simulink model "Openloop_SMA_wire_param"  (R2016b)
settings: Solver=FixedStepAuto  StartTime=0.0  StopTime=20  FixedStep=0.00001  MinStep=0.0001  RelTol=1e-3
values from neighbouring files (symbols this model uses):
  Ac = (pi*d^2)/4    (= 2.82743338823e-07)    [SMA_wire_modelling.m]    (also in ut_obs_transform.m; ut_transform.m; ut_transform_obs_param.m)
  As = 68    [Phase_Transformation_Model.m]    (also in SMA_wire_modelling.m = 0.000471238898038; ut_transform.m = 0.000471238898038; ut_transform_param.m = 0.000471238898038)
  Cp = 840    [SMA_wire_modelling.m]    (also in ut_transform.m; ut_transform_param.m)
  D = (Da+Dm)/2    (= 51500000000)    [SMA_wire_modelling.m]    (also in ut_transform.m)
  disp_i = 0.02    [SMA_wire_modelling.m]    (also in ut_obs_transform.m; ut_transform_obs_param.m)
  eps_i = disp_i/L0    (= 0.08)    [SMA_wire_modelling.m]    (also in ut_obs_transform.m; ut_transform_obs_param.m)
  eps_l = 0.067    [SMA_wire_modelling.m]    (also in ut_transform.m)
  h0 = 120    [SMA_wire_modelling.m]    (also in ut_transform.m; ut_transform_param.m)
  h2 = 0.001    [SMA_wire_modelling.m]    (also in ut_transform.m)
  Ks = 100    [SMA_wire_modelling.m]    (also in ut_obs_transform.m = real(qp_km); ut_transform.m = qp_km)
  L0 = 0.25    [SMA_wire_modelling.m]    (also in ut_obs_transform.m; ut_transform.m; ut_transform_obs_param.m; ut_transform_param.m)
  m = 1.14e-4    (= 0.000114)    [SMA_wire_modelling.m]    (also in ut_transform.m; ut_transform_param.m)
  R = 0.8491    [SMA_wire_modelling.m]
  rho_a = 8.37e-7    (= 8.37e-07)    [SMA_wire_modelling.m]    (also in ut_obs_transform.m; ut_transform_obs_param.m)
  rho_m = 9.603e-7    (= 9.603e-07)    [SMA_wire_modelling.m]    (also in ut_obs_transform.m; ut_transform_obs_param.m)
  T_amb = 20    [SMA_wire_modelling.m]    (also in ut_transform.m; ut_transform_param.m)
  theta_T = 550000    [SMA_wire_modelling.m]    (also in ut_transform.m)
  zeta0 = 1    [SMA_wire_modelling.m]    (also in zeta_dot.m)
settings Model: Creator=DAIKI  LastModifiedBy=DAIKI
settings SolverCC: InitialStep=0.0001  AlgebraicLoopSolver=LineSearch

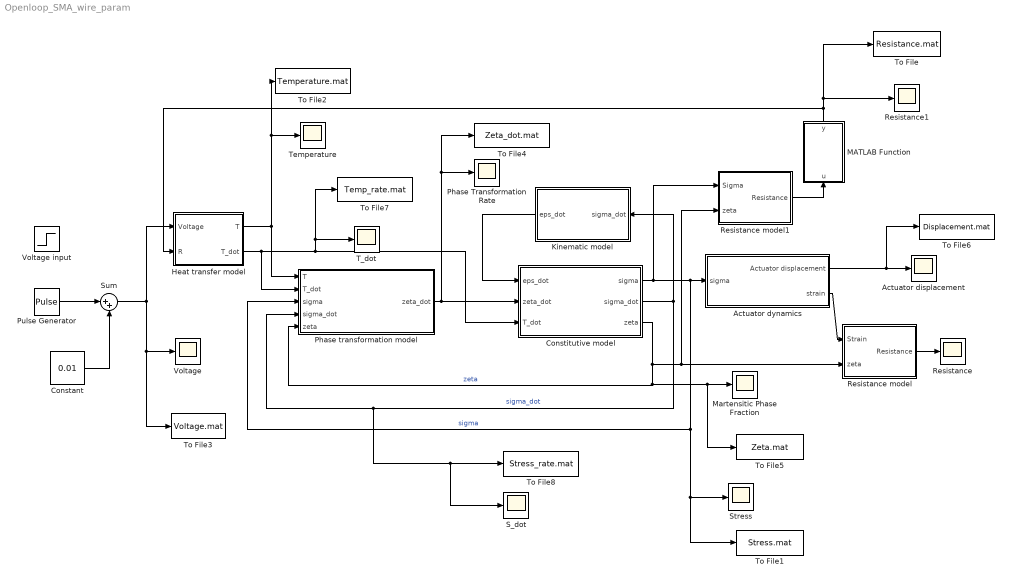
== system Openloop_SMA_wire_param ==
  Actuator displacement : Scope
  Actuator dynamics : Subsystem
  Constant : Constant  Value=0.01  VectorParams1D=off  SampleTime=-1
  Constitutive model : Subsystem
  Heat transfer model : Subsystem
  Kinematic model : Subsystem
  MATLAB Function : MATLAB Function  TreatAsAtomicUnit=on
  Martensitic Phase Fraction : Scope
  Phase Transformation Rate : Scope
  Phase transformation model : Subsystem
  Pulse Generator : DiscretePulseGenerator  PulseType=Time based  Amplitude=4  Period=40  PhaseDelay=0.5
  Resistance : Scope
  Resistance model : Subsystem
  Resistance model1 : Subsystem
  Resistance1 : Scope
  S_dot : Scope
  Stress : Scope
  Sum : Sum  Inputs=|++
  T_dot : Scope
  Temperature : Scope
  To File : ToFile  Filename=Resistance.mat  MatrixName=Res  SaveFormat=Timeseries
  To File1 : ToFile  Filename=Stress.mat  MatrixName=S  SaveFormat=Timeseries
  To File2 : ToFile  Filename=Temperature.mat  MatrixName=T  SaveFormat=Timeseries
  To File3 : ToFile  Filename=Voltage.mat  MatrixName=V  SaveFormat=Timeseries
  To File4 : ToFile  Filename=Zeta_dot.mat  MatrixName=Zeta_dot  SaveFormat=Timeseries
  To File5 : ToFile  Filename=Zeta.mat  MatrixName=Zeta  SaveFormat=Timeseries
  To File6 : ToFile  Filename=Displacement.mat  MatrixName=Dis  SaveFormat=Timeseries
  To File7 : ToFile  Filename=Temp_rate.mat  MatrixName=T_dot  SaveFormat=Timeseries
  To File8 : ToFile  Filename=Stress_rate.mat  MatrixName=S_dot  SaveFormat=Timeseries
  Voltage : Scope
  Voltage input : Step  Time=0.5  After=14  SampleTime=0
  wires:
  Actuator dynamics/1(Actuator displacement) -> To File6/1, Actuator displacement/1
  Heat transfer model/1(T) -> Phase transformation model/1(T), To File2/1, Temperature/1
  Heat transfer model/2(T_dot) -> T_dot/1, To File7/1, Constitutive model/3(T_dot), Phase transformation model/2(T_dot)
  Kinematic model/1(eps_dot) -> Constitutive model/1(eps_dot)
  Phase transformation model/1(zeta_dot) -> Constitutive model/2(zeta_dot), To File4/1, Phase Transformation Rate/1
  Constitutive model/1(sigma) -> Resistance model1/1(Sigma), To File1/1, Stress/1, Phase transformation model/3(sigma), Actuator dynamics/1(sigma)  "sigma"
  Constitutive model/2(sigma_dot) -> S_dot/1, To File8/1, Phase transformation model/4(sigma_dot), Kinematic model/1(sigma_dot)  "sigma_dot"
  Constitutive model/3(zeta) -> Resistance model1/2(zeta), Resistance model/2(zeta), To File5/1, Martensitic Phase Fraction/1, Phase transformation model/5(zeta)  "zeta"
  Actuator dynamics/2(strain) -> Resistance model/1(Strain)
  Resistance model/1(Resistance) -> Resistance/1
  Pulse Generator/1 -> Sum/1
  Constant/1 -> Sum/2
  Sum/1 -> To File3/1, Voltage/1, Heat transfer model/1(Voltage)
  Resistance model1/1(Resistance) -> MATLAB Function/1(u)
  MATLAB Function/1(y) -> Heat transfer model/2(R), Resistance1/1, To File/1

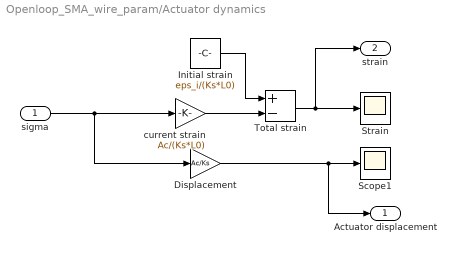
== system Openloop_SMA_wire_param/Actuator dynamics ==
  sigma : Inport
  Displacement : Gain  Gain=Ac/Ks
  Initial strain : Constant  Value=eps_i/(Ks*L0)
  Scope1 : Scope
  Strain : Scope
  Total strain : Sum  Inputs=+-
  current strain : Gain  Gain=Ac/(Ks*L0)
  Actuator displacement : Outport
  strain : Outport  Port=2
  wires:
  sigma/1 -> current strain/1, Displacement/1
  Initial strain/1 -> Total strain/1
  current strain/1 -> Total strain/2
  Total strain/1 -> strain/1, Strain/1
  Displacement/1 -> Actuator displacement/1, Scope1/1

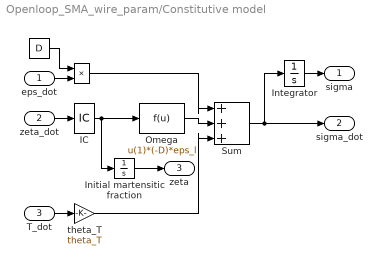
== system Openloop_SMA_wire_param/Constitutive model ==
  eps_dot : Inport
  zeta_dot : Inport  Port=2
  T_dot : Inport  Port=3
  " " : Constant  Value=D
  " " : Product  SaturateOnIntegerOverflow=on  InputSameDT=on  OutDataTypeStr=Inherit: Same as first input
  IC : InitialCondition  Value=0
  Initial martensitic fraction : Integrator  InitialCondition=zeta0  UpperSaturationLimit=1  LowerSaturationLimit=0
  Integrator : Integrator  InitialCondition=(disp_i*Ks)/Ac
  Omega : Fcn  Expr=u(1)*(-D)*eps_l
  Sum : Sum  Inputs=|+|+|+|  SaturateOnIntegerOverflow=on  InputSameDT=on  OutDataTypeStr=Inherit: Same as first input
  theta_T : Gain  Gain=theta_T  SaturateOnIntegerOverflow=on  OutDataTypeStr=Inherit: Same as input  ParamDataTypeStr=Inherit: Same as input
  sigma : Outport
  sigma_dot : Outport  Port=2
  zeta : Outport  Port=3
  wires:
  eps_dot/1 -> " "/2
  " "/1 -> " "/1
  zeta_dot/1 -> IC/1
  T_dot/1 -> theta_T/1
  IC/1 -> Initial martensitic fraction/1, Omega/1
  " "/1 -> Sum/1
  Omega/1 -> Sum/2
  theta_T/1 -> Sum/3
  Sum/1 -> Integrator/1, sigma_dot/1
  Integrator/1 -> sigma/1
  Initial martensitic fraction/1 -> zeta/1

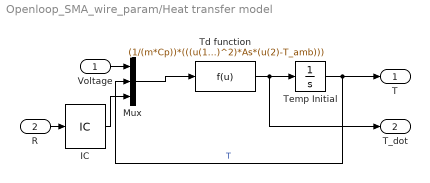
== system Openloop_SMA_wire_param/Heat transfer model ==
  Voltage : Inport
  R : Inport  Port=2
  IC : InitialCondition  Value=R
  Mux : Mux  Inputs=3
  Td function : Fcn  Expr=(1/(m*Cp))*(((u(1)^2)/u(3))-((h0+h2*u(2)^2)*As*(u(2)-T_amb)))
  Temp Initial : Integrator  InitialCondition=T_amb
  T : Outport
  T_dot : Outport  Port=2
  wires:
  Mux/1 -> Td function/1
  Voltage/1 -> Mux/1
  Temp Initial/1 -> T/1, Mux/2  "T"
  Td function/1 -> T_dot/1, Temp Initial/1
  R/1 -> IC/1
  IC/1 -> Mux/3

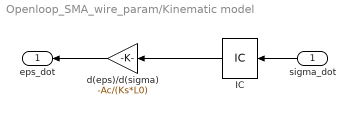
== system Openloop_SMA_wire_param/Kinematic model ==
  sigma_dot : Inport
  IC : InitialCondition  Value=0
  "d(eps)/d(sigma) " : Gain  Gain=-Ac/(Ks*L0)
  eps_dot : Outport
  wires:
  "d(eps)/d(sigma) "/1 -> eps_dot/1
  sigma_dot/1 -> IC/1
  IC/1 -> "d(eps)/d(sigma) "/1

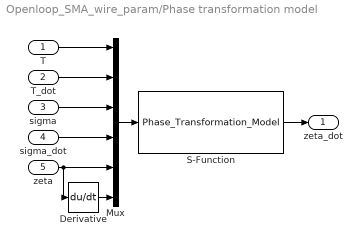
== system Openloop_SMA_wire_param/Phase transformation model ==
  T : Inport
  T_dot : Inport  Port=2
  sigma : Inport  Port=3
  sigma_dot : Inport  Port=4
  zeta : Inport  Port=5
  Derivative : Derivative
  Mux : Mux  Inputs=6
  S-Function : S-Function  FunctionName=Phase_Transformation_Model  SFunctionDeploymentMode=off  EnableBusSupport=off
  zeta_dot : Outport
  wires:
  sigma/1 -> Mux/3
  T_dot/1 -> Mux/2
  T/1 -> Mux/1
  sigma_dot/1 -> Mux/4
  Mux/1 -> S-Function/1
  S-Function/1 -> zeta_dot/1
  Derivative/1 -> Mux/6
  zeta/1 -> Mux/5, Derivative/1

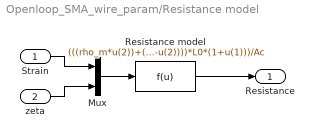
== system Openloop_SMA_wire_param/Resistance model ==
  Strain : Inport
  zeta : Inport  Port=2
  Mux : Mux  Inputs=2
  Resistance model : Fcn  Expr=(((rho_m*u(2))+(rho_a*(1-u(2))))*L0*(1+u(1)))/Ac
  Resistance : Outport
  wires:
  Resistance model/1 -> Resistance/1
  Mux/1 -> Resistance model/1
  Strain/1 -> Mux/1
  zeta/1 -> Mux/2

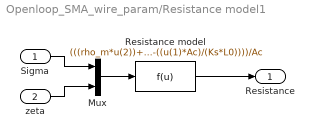
== system Openloop_SMA_wire_param/Resistance model1 ==
  Sigma : Inport
  zeta : Inport  Port=2
  Mux : Mux  Inputs=2
  Resistance model : Fcn  Expr=(((rho_m*u(2))+((1-u(2))*rho_a))*L0*(1+eps_i-((u(1)*Ac)/(Ks*L0))))/Ac
  Resistance : Outport
  wires:
  Resistance model/1 -> Resistance/1
  Mux/1 -> Resistance model/1
  Sigma/1 -> Mux/1
  zeta/1 -> Mux/2

== matlab function Openloop_SMA_wire_param/MATLAB Function ==
  data: u input; y output
function y = fcn(u)

percent = 0.0001;
low = (-0.8491)*(percent/100);
high = (0.8491)*(percent/100);

w = low + (high-low)*rand(1,1);
y = u + w;
